simulink model "lacze2"  (Simulink 4.00)
settings: Solver=ode45  StartTime=0  StopTime=1  RelTol=1e-3
libraries: commanapbnd2 x6, dspstat3 x3, dsparch3 x2, commsource2 x1
settings Model: LimitDataPoints=off  MaxDataPoints=10000  RTWOptions="-aEnforceIntegerDowncast=1 -aExtMode=0 -aFoldNonRolledExpr=1 -aForceParamTrailComments=0 -aGenerateComments=1 -aIgnoreCustomStorageClasses=1 -aIncHierarchyInIds=0 -aInlineInvariantSignals=0 -aLocalBlockOutputs=1 -aLogVarNameModifier=\"rt_\" -aRTWVerbose=1 -aRollThreshold=5 -aShowEliminatedStatements=1"  BlockReductionOpt=off

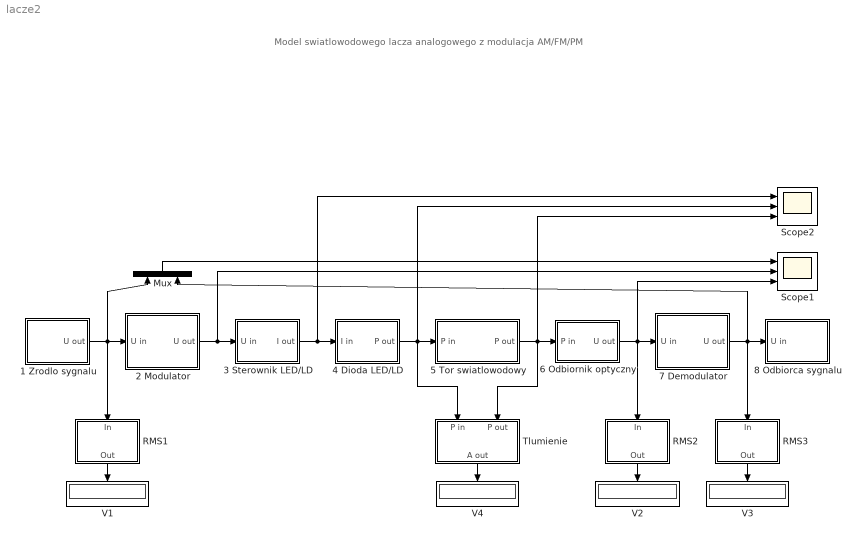
== system lacze2 ==
  note: Model swiatlowodowego lacza analogowego z modulacja AM/FM/PM
  1 Zrodlo sygnalu : Subsystem  mask(Źródło sygnału){Asyg=1, fsyg=2}
      mask prompts: Asyg "Amplituda sygnału [V]:"; fsyg "Częstotliwość sygnału [MHz]:"
      mask help:
      | Generuje sinusoidalny sygnał o określonej amplitudzie i częstotliowości. Wartość amplitudy wyrażona jest w V i nie powinna przekraczać 10 V.
      | W przypadku podania większej wartości, zostanie ona ograniczona
      | do 10 V.
      |
      | Częstotliwość sygnału wyrażona jest w MHz i dla poprawności dokonywanej modulacji powinna stanowić ok. 1/10 częstotliwości nośnej która może wynosić 200, 400, 600 lub 800 MHz.
      settings: RTWFcnNameOpts=Auto  RTWFileNameOpts=Auto
      mask Help: No help
      mask Display: disp('Sygnal\nnadawany')
  2 Modulator : Subsystem  mask(Modulator AM/FM/PM){modulacja=AM, nosna=200, czulosc=1}
      mask prompts: modulacja "Rodzaj modulacji:"; nosna "Częstotliwość nośnej [MHz]:"; czulosc "Czułość modulacji AM [1/V], FM [MHz/V], PM [rad/V]:"
      mask help:
      | Dokonuje operacji modulacji (w zależności od wyboru AM/FM/PM) sygnałem podanym na wejście. Wartość amplitudy nośnej jest stała i wynosi Ac = 1 V.
      |
      | Częstotliwość nośnej należy dobrać mając na uwadze częstotliwość sygnału przesylanego.
      |
      | Należy określić czułość modulatora.
      | W przypadku modulacji AM - ka [1/V]. Głębokość modulacji m zależy od amplitudy sygnału wejściowego Uin oraz od czułości i wynosi:
      |
      | m = ka * Uin * 100%
      |
      | Dla modulacji FM i PM są określane odpowiednio: czułość częstotliwościowa - kf [MHz/V] i czułość fazowa - kp [rad/V].
      mask init:
      | if (nosna == 1)
      | fnos = 100;
      | ikona2 = ['       ';'       ';'       ';'100 MHz'];
      | elseif (nosna == 2)
      | fnos = 200;
      | ikona2 = ['       ';'       ';'       ';'200 MHz'];
      | elseif (nosna == 3)
      | fnos = 400;
      | ikona2 = ['       ';'       ';'       ';'400 MHz'];
      | else
      | fnos = 800;
      | ikona2 = ['       ';'       ';'       ';'800 MHz'];
      | end;
      | 
      | if (modulacja == 1)
      | ikona1 = ['  ';'AM'];
      | elseif (modulacja == 2)
      | ikona1 = ['  ';'FM'];
      | else
      | ikona1 = ['  ';'PM'];
      | end;
      settings: RTWFcnNameOpts=Auto  RTWFileNameOpts=Auto
      mask Help: No help
      mask StyleString: popup(AM|FM|PM),popup(100|200|400|800),edit
      mask Display:
      | disp('Modulator\n\n')
      | disp(ikona1)
      | disp(ikona2)
  3 Sterownik LED/LD : Subsystem  mask(Sterownik diody LED/Lasera){K1=10, Ipol=80, Iogr=100}
      mask prompts: K1 "Czułość prądowa sterownika [mA/V]:"; Ipol "Prąd polaryzacji wstępnej [mA]:"; Iogr "Ograniczenie prądu maksymalnego diody LED/LD [mA]:"
      mask help:
      | Ma za zadanie wysterowanie diody LED lub lasera sygnałem prądowym. Wejście sterownika jest napięciowe. Należy podać czułość prądową sterownika oraz prąd polaryzacji wstępnej uwzględniając parametry nadajnika optycznego.
      |
      | Wartość ograniczenia prądu maksymalnego diody należy wprowadzić
      | w celu zabezpieczenia diody LED lub lasera przed uszkodzeniem.
      | W przypadku gdy sygnał przekroczy wartość dopuszczalną, zadziała ogranicznik prądu.
      settings: RTWFcnNameOpts=Auto  RTWFileNameOpts=Auto
      mask Help: No help
      mask Display: disp('Sterownik\ndiody')
  4 Dioda LED/LD : Subsystem  mask(Dioda LED/Laser){dioda=Laser-2}
      mask prompts: dioda "Typ zastosowanej diody"
      mask help:
      | Przetwarza prąd wejściowy na moc optyczną. Blok obejmuje nadajnik optyczny zintegrowany ze sprzęgaczem wejściowym. Do wyboru są
      | dwie diody LED oraz dwa lasery. Parametry źródeł światła podane są
      | w tabeli:
      |                          Imax            Pmax         Iprog
      | |-------------------|------------------|------------------|-----------------|
      | |    LED-1     |     80 mA   |   0.1 mW   |     0 mA    |
      | |    LED-2     |   140 mA   |   0.5 mW   |     0 mA    |
      | |    Laser-1   |   120 mA   |   1.0 mW   |    40 mA   |
      | |    Laser-2   |   100 mA   |   2.0 mW   |    60 mA   |
      | ----------------------------------------------------------------------------
      | W przypadku przekroczenia prądu maksymalnego diody lub lasera element ulega uszkodzeniu i przestaje generować sygnał optyczny.
      mask init:
      | Baza_Imax = [80 140 120 100];
      | Baza_Pmax = [0.1 0.5 1 2];
      | Baza_Iprog = [0 0 40 60];
      | K2 = Baza_Pmax(dioda) / (Baza_Imax(dioda) - Baza_Iprog(dioda));
      | Imax = Baza_Imax(dioda);
      | Iprog = Baza_Iprog(dioda);
      | 
      | if (dioda == 1)
      | ikona = ['LED-1'];
      | elseif (dioda == 2)
      | ikona = ['LED-2'];
      | elseif (dioda == 3)
      | ikona = ['Laser-1'];
      | else
      | ikona = ['Laser-2'];
      | end;
      settings: RTWFcnNameOpts=Auto  RTWFileNameOpts=Auto
      mask Help: No help
      mask StyleString: popup(LED-1|LED-2|Laser-1|Laser-2)
      mask Display: disp(ikona)
  5 Tor swiatlowodowy : Subsystem  mask(Tor światłowodowy){lf=36, Af=0.5, n=5, Ls=0.2, m=2, Lm=0.5}
      mask prompts: lf "Długość światłowodu - lf [km]:"; Af "Tłumienie jednostkowe - Af [dB/km]:"; n "Ilość połączeń spawanych - n:"; Ls "Tłumienie połączenia spawanego - Ls [dB]:"; m "Ilość połączeń rozłącznych - m:"; Lm "Tłumienie połączenia rozłącznego - Lm [dB]:"
      mask help:
      | Tłumi sygnał wejściowy o wartość określoną przez parametry. Wartość tłumienia całkowitego wynosi:
      |
      | A(dB) = (-1) * (Af * lf + Ls * n + Lm * m)
      settings: RTWFcnNameOpts=Auto  RTWFileNameOpts=Auto
      mask Display: disp('Tor\nswiatlowodowy')
  6 Odbiornik optyczny : Subsystem  mask(Odbiornik optyczny){K3=0.2, szum=off}
      mask prompts: K3 "Czułość odbiornika [V/uW]:"; szum "Pomiar wartości szumu"
      mask help:
      | Obejmuje sprzęgacz optyczny zintegrowany z detektorem optycznym
      | i wzmacniaczem transimpedancyjnym. Przetwarza moc optyczną na sygnał napięciowy oraz eliminuje składowa stałą zawartą w sygnale optycznym (sygnał ze składową stałą nie daje się prawidłowo demodulować). Należy podać czułość odbiornika.
      |
      | Zaznaczenie funkcji "Pomiar wartości szumu" powoduje odłączenie mocy optycznej od wejścia i umożliwia pomiar wartości szumu generowanego przez odbiornik. Aby obliczyć moc szumu należy uwzględnić czułość odbiornika.
      mask init:
      | szum = szum + 1;
      | Unas = 5;
      settings: RTWFcnNameOpts=Auto  RTWFileNameOpts=Auto
      mask Help: No Help
      mask Display: disp('Odbiornik\noptyczny')
  7 Demodulator : Subsystem  mask(Demodulator AM/FM/PM){modulacja=AM, nosna=200, czulosc=1, filtr=off, szum=off}
      mask prompts: modulacja "Rodzaj modulacji:"; nosna "Częstotliwość nośnej [MHz]:"; czulosc "Czułość modulacji AM [1/V], FM [MHz/V], PM [rad/V]:"; filtr "Dodatkowy filtr nośnej"; szum "Pomiar wartości szumu"
      mask help:
      | Dokonuje operacji demodulacji (w zależności od wyboru AM/FM/PM) sygnału podanego na wejście. Wartość amplitudy nośnej jest stała i wynosi Ac = 1 V. Daltego w przypadku demodulacji AM należy pamiętać o odpowiednim ustawieniu czułości odbiornika optycznego, tak aby średnia amplituda nośnej wynosiła ok. 1 V.
      |
      | Wartości częstotliwości nośnej i czułości modulacji należy podać takie same jak w modulatorze. W przeciwnym wypadku fala zdemodulowana będzie zniekształcona.
      |
      | Zaznaczenie funkcji "Dodatkowy filtr nośnej" powoduje załączenie filtru dolnoprzepustowego eliminującego pozostałości nośnej.
      |
      | Funkcja "Pomiar wartości szumu" powinna być zaznaczona przy pomiarze szumu.
      mask init:
      | filtr = filtr + 1;
      | 
      | if (nosna == 1)
      | fnos = 100;
      | ikona2 = ['       ';'       ';'       ';'100 MHz'];
      | elseif (nosna == 2)
      | fnos = 200;
      | ikona2 = ['       ';'       ';'       ';'200 MHz'];
      | elseif (nosna == 3)
      | fnos = 400;
      | ikona2 = ['       ';'       ';'       ';'400 MHz'];
      | else
      | fnos = 800;
      | ikona2 = ['       ';'       ';'       ';'800 MHz'];
      | end;
      | 
      | if (modulacja == 1)
      | ikona1 = ['  ';'AM'];
      | elseif (modulacja == 2)
      | ikona1 = ['  ';'FM'];
      | else
      | ikona1 = ['  ';'PM'];
      | end;
      settings: RTWFcnNameOpts=Auto  RTWFileNameOpts=Auto
      mask Help: No help.
      mask StyleString: popup(AM|FM|PM),popup(100|200|400|800),edit,checkbox,checkbox
      mask Display:
      | disp('Demodulator\n\n')
      | disp(ikona1)
      | disp(ikona2)
  8 Odbiorca sygnalu : Subsystem
      settings: RTWFcnNameOpts=Auto  RTWFileNameOpts=Auto
      mask Type: Odbiorca sygnału
      mask Description: Odbiera sygnał przesylany od nadawcy.
      mask Help: No help
      mask Display: disp('Sygnal\nodbierany')
  Mux : Mux  Orientation=up  Inputs=2
  RMS1 : Subsystem  Orientation=down
      settings: RTWFcnNameOpts=Auto  RTWFileNameOpts=Auto
      mask Type: Pomiar RMS
      mask Description: Oblicza wartość skuteczną sygnału po zakończeniu symulacji.
      mask Display: disp('RMS')
  RMS2 : Subsystem  Orientation=down
      settings: RTWFcnNameOpts=Auto  RTWFileNameOpts=Auto
      mask Type: Pomiar RMS
      mask Description: Oblicza wartość skuteczną sygnału po zakończeniu symulacji.
      mask Display: disp('RMS')
  RMS3 : Subsystem  Orientation=down
      settings: RTWFcnNameOpts=Auto  RTWFileNameOpts=Auto
      mask Type: Pomiar RMS
      mask Description: Oblicza wartość skuteczną sygnału po zakończeniu symulacji.
      mask Display: disp('RMS')
  Scope1 : Scope  NumInputPorts=3
      settings: TimeRange=auto  YMin=-2.5~-2.5~-2.5  YMax=2.5~2.5~2.5  SaveToWorkspace=off  SaveName=ScopeData  DataFormat=Array  MaxDataPoints=10000
  Scope2 : Scope  NumInputPorts=3
      settings: TimeRange=auto  YMin=-5~-0.25~-2.5  YMax=125~2.25~22.5  SaveToWorkspace=off  DataFormat=Array  MaxDataPoints=10000
  Tlumienie : Subsystem  Orientation=down  mask(Przetwornik do pomiaru tłumienia){tlumienie=dB}
      mask prompts: tlumienie "Pomiar tłumienia:"
      mask help: Podając na wejścia przetwornika sygnały z wejścia i wyjścia światłowodu uzyskuje się wartość tłumienia całkowitego toru światłowodowego wyrażoną, w zależności od wyboru, w dB lub uW/uW.
      mask init:
      | if (tlumienie == 1)
      | ikona = ['  ';'  ';'dB'];
      | else
      | ikona = ['     ';'     ';'uW/uW'];
      | end;
      settings: RTWFcnNameOpts=Auto  RTWFileNameOpts=Auto
      mask StyleString: popup(dB|uW/uW)
      mask Display:
      | disp('Tlumienie\n')
      | disp(ikona)
  V{1..4} (4 alike) : Display
      settings: Orientation=down  Format=short
  wires:
  3 Sterownik LED/LD/1(I out) -> 4 Dioda LED/LD/1(I in), Scope2/1
  1 Zrodlo sygnalu/1(U out) -> 2 Modulator/1(U in), RMS1/1(In), Mux/1
  5 Tor swiatlowodowy/1(P out) -> 6 Odbiornik optyczny/1(P in), Tlumienie/2(P out), Scope2/3
  2 Modulator/1(U out) -> 3 Sterownik LED/LD/1(U in), Scope1/2
  6 Odbiornik optyczny/1(U out) -> 7 Demodulator/1(U in), RMS2/1(In), Scope1/3
  4 Dioda LED/LD/1(P out) -> 5 Tor swiatlowodowy/1(P in), Tlumienie/1(P in), Scope2/2
  RMS1/1(Out) -> V1/1
  RMS2/1(Out) -> V2/1
  7 Demodulator/1(U out) -> RMS3/1(In), 8 Odbiorca sygnalu/1(U in), Mux/2
  RMS3/1(Out) -> V3/1
  Tlumienie/1(A out) -> V4/1
  Mux/1 -> Scope1/1

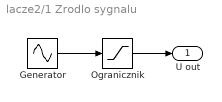
== system lacze2/1 Zrodlo sygnalu ==
  Generator : Sin  SineType=Time-based  Amplitude=Asyg  Bias=0  Frequency=2*pi*fsyg  Phase=0  Samples=10  SampleTime=0  Offset=0
  Ogranicznik : Saturate  UpperLimit=10  LowerLimit=-10  LinearizeAsGain=on
  U out : Outport  Port=1
  wires:
  Generator/1 -> Ogranicznik/1
  Ogranicznik/1 -> U out/1

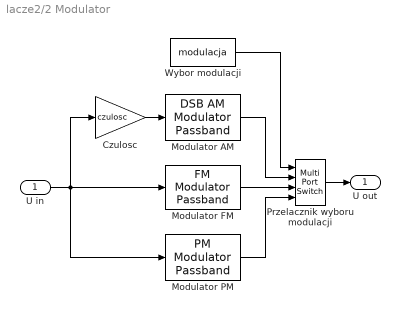
== system lacze2/2 Modulator ==
  U in : Inport  Port=1  LatchInput=off
  Czulosc : Gain  Gain=czulosc  Multiplication=Element-wise(K.*u)  SaturateOnIntegerOverflow=on
  Modulator AM : commanapbnd2/DSB AM Modulator Passband  Fc=fnos  Ph=0  Offset=1
  Modulator FM : commanapbnd2/FM Modulator Passband  Fc=fnos  Ph=0  HzPerV=czulosc  ts=0.1/fnos  td=Inf
  Modulator PM : commanapbnd2/PM Modulator Passband  Fc=fnos  Ph=0  Kc=czulosc  td=Inf
  Przelacznik wyboru modulacji : MultiPortSwitch  Inputs=3
  Wybor modulacji : Constant  Value=modulacja
  U out : Outport  Port=1
  wires:
  Modulator AM/1 -> Przelacznik wyboru modulacji/2
  Modulator FM/1 -> Przelacznik wyboru modulacji/3
  Modulator PM/1 -> Przelacznik wyboru modulacji/4
  Wybor modulacji/1 -> Przelacznik wyboru modulacji/1
  Przelacznik wyboru modulacji/1 -> U out/1
  U in/1 -> Modulator FM/1, Modulator PM/1, Czulosc/1
  Czulosc/1 -> Modulator AM/1

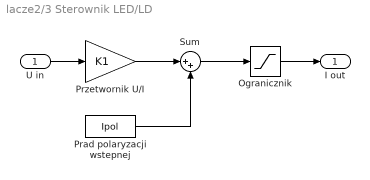
== system lacze2/3 Sterownik LED/LD ==
  U in : Inport  Port=1  LatchInput=off
  Ogranicznik : Saturate  UpperLimit=Iogr  LowerLimit=0  LinearizeAsGain=on
  Prad polaryzacji wstepnej : Constant  Value=Ipol
  Przetwornik U/I : Gain  Gain=K1  Multiplication=Element-wise(K.*u)  SaturateOnIntegerOverflow=on
  Sum : Sum  Inputs=|++  SaturateOnIntegerOverflow=on
  I out : Outport  Port=1
  wires:
  Przetwornik U/I/1 -> Sum/1
  Prad polaryzacji wstepnej/1 -> Sum/2
  Sum/1 -> Ogranicznik/1
  U in/1 -> Przetwornik U/I/1
  Ogranicznik/1 -> I out/1

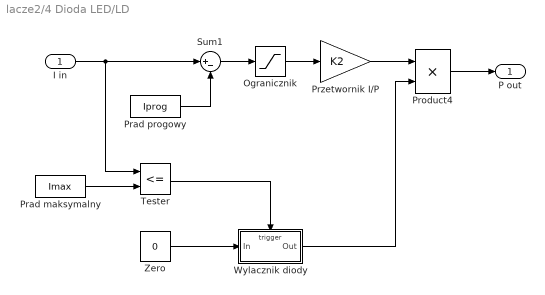
== system lacze2/4 Dioda LED/LD ==
  I in : Inport  Port=1  LatchInput=off
  Ogranicznik : Saturate  UpperLimit=inf  LowerLimit=0  LinearizeAsGain=on
  Prad maksymalny : Constant  Value=Imax
  Prad progowy : Constant  Value=Iprog
  Product4 : Product  Inputs=2  Multiplication=Element-wise(.*)  SaturateOnIntegerOverflow=on
  Przetwornik I/P : Gain  Gain=K2  Multiplication=Element-wise(K.*u)  SaturateOnIntegerOverflow=on
  Sum1 : Sum  Inputs=|+-  SaturateOnIntegerOverflow=on
  Tester : RelationalOperator  Operator=<=
  Wylacznik diody : Subsystem  TreatAsAtomicUnit=on
      settings: RTWFcnNameOpts=Auto  RTWFileNameOpts=Auto
  Zero : Constant  Value=0
  P out : Outport  Port=1
  wires:
  Prad progowy/1 -> Sum1/2
  Sum1/1 -> Ogranicznik/1
  Ogranicznik/1 -> Przetwornik I/P/1
  I in/1 -> Sum1/1, Tester/1
  Przetwornik I/P/1 -> Product4/1
  Product4/1 -> P out/1
  Tester/1 -> Wylacznik diody/Trigger
  Wylacznik diody/1(Out) -> Product4/2
  Zero/1 -> Wylacznik diody/1(In)
  Prad maksymalny/1 -> Tester/2

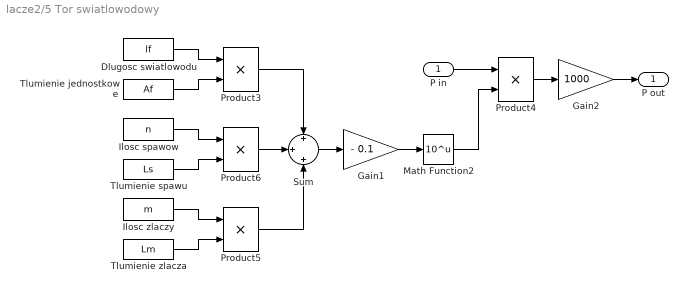
== system lacze2/5 Tor swiatlowodowy ==
  P in : Inport  Port=1  LatchInput=off
  Dlugosc swiatlowodu : Constant  Value=lf
  Gain1 : Gain  Gain=- 0.1  Multiplication=Element-wise(K.*u)  SaturateOnIntegerOverflow=on
  Gain2 : Gain  Gain=1000  Multiplication=Element-wise(K.*u)  SaturateOnIntegerOverflow=on
  Ilosc spawow : Constant  Value=n
  Ilosc zlaczy : Constant  Value=m
  Math Function2 : Math  Operator=10^u  OutputSignalType=auto
  Product{3..6} (4 alike) : Product  Inputs=2  Multiplication=Element-wise(.*)  SaturateOnIntegerOverflow=on
  Sum : Sum  Inputs=+|+|+  SaturateOnIntegerOverflow=on
  Tlumienie jednostkowe : Constant  Value=Af
  Tlumienie spawu : Constant  Value=Ls
  Tlumienie zlacza : Constant  Value=Lm
  P out : Outport  Port=1
  wires:
  Math Function2/1 -> Product4/2
  Product4/1 -> Gain2/1
  Dlugosc swiatlowodu/1 -> Product3/1
  Tlumienie jednostkowe/1 -> Product3/2
  Sum/1 -> Gain1/1
  Gain1/1 -> Math Function2/1
  Product3/1 -> Sum/1
  P in/1 -> Product4/1
  Ilosc zlaczy/1 -> Product5/1
  Tlumienie zlacza/1 -> Product5/2
  Ilosc spawow/1 -> Product6/1
  Tlumienie spawu/1 -> Product6/2
  Product6/1 -> Sum/2
  Product5/1 -> Sum/3
  Gain2/1 -> P out/1

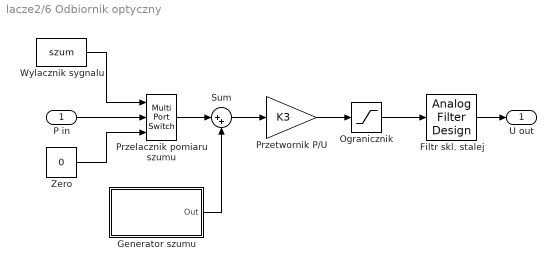
== system lacze2/6 Odbiornik optyczny ==
  P in : Inport  Port=1  LatchInput=off
  Filtr skl. stalej : dsparch3/Analog Filter Design  method=Butterworth  filttype=Highpass  N=1  Wlo=2*pi*50  Whi=80  Rp=2  Rs=40
  Generator szumu : Subsystem  mask(Generator szumu){Pszum=0.1}
      mask prompts: Pszum "Moc szumu [uW]:"
      settings: RTWFcnNameOpts=Auto  RTWFileNameOpts=Auto
      mask Display:
      | plot(0,0,100,100,[95 5 10 10 10 (100-15)*[0:1/30:1]+10],[75 75 75 70 95 randn(1,31)*10+75]);
      | disp('\nGenerator szumu')
  Ogranicznik : Saturate  UpperLimit=Unas  LowerLimit=-Unas  LinearizeAsGain=on
  Przelacznik pomiaru szumu : MultiPortSwitch  Inputs=2
  Przetwornik P/U : Gain  Gain=K3  Multiplication=Element-wise(K.*u)  SaturateOnIntegerOverflow=on
  Sum : Sum  Inputs=|++  SaturateOnIntegerOverflow=on
  Wylacznik sygnalu : Constant  Value=szum
  Zero : Constant  Value=0
  U out : Outport  Port=1
  wires:
  Przetwornik P/U/1 -> Ogranicznik/1
  Sum/1 -> Przetwornik P/U/1
  Generator szumu/1(Out) -> Sum/2
  Ogranicznik/1 -> Filtr skl. stalej/1
  Wylacznik sygnalu/1 -> Przelacznik pomiaru szumu/1
  P in/1 -> Przelacznik pomiaru szumu/2
  Przelacznik pomiaru szumu/1 -> Sum/1
  Zero/1 -> Przelacznik pomiaru szumu/3
  Filtr skl. stalej/1 -> U out/1

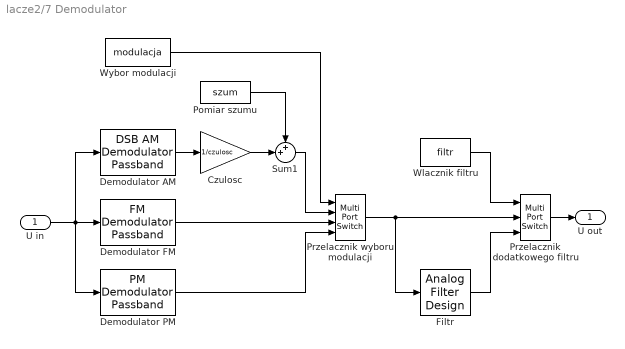
== system lacze2/7 Demodulator ==
  U in : Inport  Port=1  LatchInput=off
  Czulosc : Gain  Gain=1/czulosc  Multiplication=Element-wise(K.*u)  SaturateOnIntegerOverflow=on
  Demodulator AM : commanapbnd2/DSB AM Demodulator Passband  Fc=fnos  Ph=0  num=[0.0201 0.0402 0.0201]  den=[1.0000 -1.5610 0.6414]  ts=0.1/fnos  Offset=1
  Demodulator FM : commanapbnd2/FM Demodulator Passband  Fc=fnos  Ph=0  HzPerVolt=czulosc  num=[0.0201 0.0402 0.0201]  den=[1.0000 -1.5610 0.6414]  ts=0.1/fnos
  Demodulator PM : commanapbnd2/PM Demodulator Passband  Fc=fnos  Ph=0  Kc=czulosc  num=[0.0201 0.0402 0.0201]  den=[1.0000 -1.5610 0.6414]  HzPerVolt=1  ts=0.1/fnos
  Filtr : dsparch3/Analog Filter Design  method=Butterworth  filttype=Lowpass  N=2  Wlo=2*pi*0.5*fnos  Whi=80  Rp=2  Rs=40
  Pomiar szumu : Constant  Value=szum
  Przelacznik dodatkowego filtru : MultiPortSwitch  Inputs=2
  Przelacznik wyboru modulacji : MultiPortSwitch  Inputs=3
  Sum1 : Sum  Inputs=++|  SaturateOnIntegerOverflow=on
  Wlacznik filtru : Constant  Value=filtr
  Wybor modulacji : Constant  Value=modulacja
  U out : Outport  Port=1
  wires:
  Demodulator AM/1 -> Czulosc/1
  Demodulator FM/1 -> Przelacznik wyboru modulacji/3
  Demodulator PM/1 -> Przelacznik wyboru modulacji/4
  Wybor modulacji/1 -> Przelacznik wyboru modulacji/1
  U in/1 -> Demodulator FM/1, Demodulator AM/1, Demodulator PM/1
  Przelacznik dodatkowego filtru/1 -> U out/1
  Przelacznik wyboru modulacji/1 -> Przelacznik dodatkowego filtru/2, Filtr/1
  Filtr/1 -> Przelacznik dodatkowego filtru/3
  Wlacznik filtru/1 -> Przelacznik dodatkowego filtru/1
  Sum1/1 -> Przelacznik wyboru modulacji/2
  Pomiar szumu/1 -> Sum1/1
  Czulosc/1 -> Sum1/2

== system lacze2/8 Odbiorca sygnalu ==
  U in : Inport  Port=1  LatchInput=off
  Odbiorca : Terminator
  wires:
  U in/1 -> Odbiorca/1

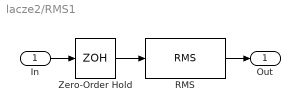
== system lacze2/RMS1 ==
  In : Inport  Port=1  LatchInput=off
  RMS : dspstat3/RMS  run=on  reset_popup=None
  Zero-Order Hold : ZeroOrderHold  SampleTime=0.0001
  Out : Outport  Port=1
  wires:
  Zero-Order Hold/1 -> RMS/1
  In/1 -> Zero-Order Hold/1
  RMS/1 -> Out/1

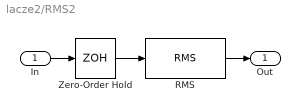
== system lacze2/RMS2 ==
  In : Inport  Port=1  LatchInput=off
  RMS : dspstat3/RMS  run=on  reset_popup=None
  Zero-Order Hold : ZeroOrderHold  SampleTime=0.0001
  Out : Outport  Port=1
  wires:
  Zero-Order Hold/1 -> RMS/1
  In/1 -> Zero-Order Hold/1
  RMS/1 -> Out/1

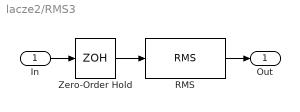
== system lacze2/RMS3 ==
  In : Inport  Port=1  LatchInput=off
  RMS : dspstat3/RMS  run=on  reset_popup=None
  Zero-Order Hold : ZeroOrderHold  SampleTime=0.0001
  Out : Outport  Port=1
  wires:
  Zero-Order Hold/1 -> RMS/1
  In/1 -> Zero-Order Hold/1
  RMS/1 -> Out/1

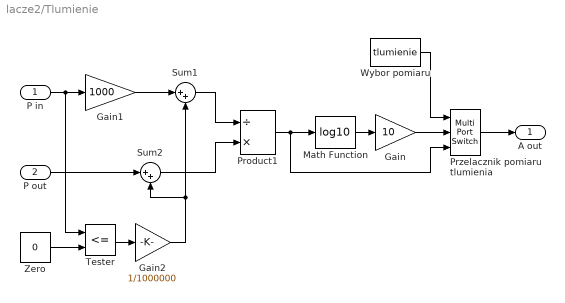
== system lacze2/Tlumienie ==
  P in : Inport  Port=1  LatchInput=off
  P out : Inport  Port=2  LatchInput=off
  Gain : Gain  Gain=10  Multiplication=Element-wise(K.*u)  SaturateOnIntegerOverflow=on
  Gain1 : Gain  Gain=1000  Multiplication=Element-wise(K.*u)  SaturateOnIntegerOverflow=on
  Gain2 : Gain  Gain=1/1000000  Multiplication=Element-wise(K.*u)  SaturateOnIntegerOverflow=on
  Math Function : Math  Operator=log10  OutputSignalType=auto
  Product1 : Product  Inputs=/*  Multiplication=Element-wise(.*)  SaturateOnIntegerOverflow=on
  Przelacznik pomiaru tlumienia : MultiPortSwitch  Inputs=2
  Sum1 : Sum  Inputs=|++  SaturateOnIntegerOverflow=on
  Sum2 : Sum  Inputs=|++  SaturateOnIntegerOverflow=on
  Tester : RelationalOperator  Operator=<=
  Wybor pomiaru : Constant  Value=tlumienie
  Zero : Constant  Value=0
  A out : Outport  Port=1
  wires:
  P in/1 -> Gain1/1, Tester/1
  Product1/1 -> Math Function/1, Przelacznik pomiaru tlumienia/3
  Wybor pomiaru/1 -> Przelacznik pomiaru tlumienia/1
  Math Function/1 -> Gain/1
  Gain/1 -> Przelacznik pomiaru tlumienia/2
  Sum1/1 -> Product1/1
  Sum2/1 -> Product1/2
  Gain1/1 -> Sum1/1
  Tester/1 -> Gain2/1
  Zero/1 -> Tester/2
  Przelacznik pomiaru tlumienia/1 -> A out/1
  P out/1 -> Sum2/1
  Gain2/1 -> Sum1/2, Sum2/2

== system lacze2/4 Dioda LED/LD/Wylacznik diody ==
  In : Inport  Port=1  LatchInput=off
  Trigger : TriggerPort  TriggerType=falling  OutputDataType=auto
  Out : Outport  Port=1  InitialOutput=1
  wires:
  In/1 -> Out/1

== system lacze2/6 Odbiornik optyczny/Generator szumu ==
  Generator szumu : commsource2/Gaussian Noise Generator  m=0  d=0.5  s=54321  Ts=0.0001  frameBased=off  sampPerFrame=1  orient=off
  Przetwornik P/U1 : Gain  Gain=1.39*Pszum  Multiplication=Element-wise(K.*u)  SaturateOnIntegerOverflow=on
  Out : Outport  Port=1
  wires:
  Generator szumu/1 -> Przetwornik P/U1/1
  Przetwornik P/U1/1 -> Out/1
